simulink model "CurrentSystem2019a"  (R2019a)
settings: Solver=ode23tb  StartTime=0  StopTime=24*365*60*60  RelTol=0.1  EnableMultiTasking=on
PreLoadFcn:
  | power_13NodeTestFeeder_init;
undefined symbols (not defined in the file): ABSOLARCap, ABWindCap, BCSOLARCap, BCWindCap, C_601, C_602, C_603, C_604, C_605, C_606, C_607, ft2km, L_601, L_602, L_603, L_604, L_605, L_606, L_607, MBSOLARCap, MBWindCap, NBSOLARCap, NBWindCap, NLSOLARCap, NLWindCap, NSSOLARCap, NSWindCap, NTSOLARCap, NTWindCap, NUSOLARCap, NUWindCap, ONSOLARCap, ONWindCap, PEISOLARCap, PEIWindCap, QCSOLARCap, QCWindCap, R_601, R_602, R_603, R_604, R_605, R_606, R_607, SKSOLARCap, SKWindCap, T_Disconnect, T_Reconnect, Yearsec, YTSOLARCap, YTWindCap
libraries: powerlib_meascontrol x70, powerlib x67, sps_avr x1, spsDieselMotorModel x1
(part 3 of 3)

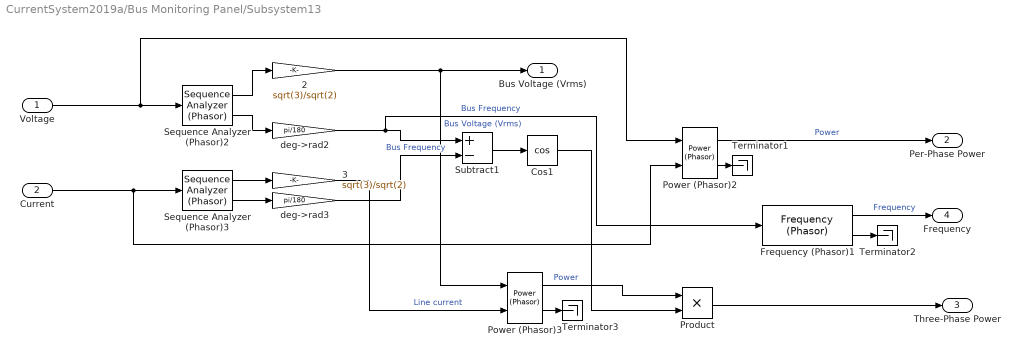
== system CurrentSystem2019a/Bus Monitoring Panel/Subsystem13 ==
  Voltage : Inport
  Current : Inport  Port=2
  " 2" : Gain  Gain=sqrt(3)/sqrt(2)
  " 3" : Gain  Gain=sqrt(3)/sqrt(2)
  Cos1 : Trigonometry  Operator=cos
  Frequency (Phasor)1 : powerlib_meascontrol/Measurements/Frequency (Phasor)  Fn=60  T=0.1
      settings: SourceProductName=Simscape Electrical  SourceProductBaseCode=PS
  Power (Phasor)2 : powerlib_meascontrol/Measurements/Power (Phasor)
      settings: SourceProductName=Simscape Electrical  SourceProductBaseCode=PS
  Power (Phasor)3 : powerlib_meascontrol/Measurements/Power (Phasor)
      settings: SourceProductName=Simscape Electrical  SourceProductBaseCode=PS
  Product : Product
  Sequence Analyzer (Phasor)2 : powerlib_meascontrol/Measurements/Sequence Analyzer (Phasor)  seq=Positive
      settings: SourceProductName=Simscape Electrical  SourceProductBaseCode=PS
  Sequence Analyzer (Phasor)3 : powerlib_meascontrol/Measurements/Sequence Analyzer (Phasor)  seq=Positive
      settings: SourceProductName=Simscape Electrical  SourceProductBaseCode=PS
  Subtract1 : Sum  Inputs=+-
  Terminator1 : Terminator
  Terminator2 : Terminator
  Terminator3 : Terminator
  deg->rad2 : Gain  Gain=pi/180
  deg->rad3 : Gain  Gain=pi/180
  Bus Voltage (Vrms) : Outport  VectorParamsAs1DForOutWhenUnconnected=on
  Per-Phase Power : Outport  Port=2  VectorParamsAs1DForOutWhenUnconnected=on
  Three-Phase Power : Outport  Port=3  VectorParamsAs1DForOutWhenUnconnected=on
  Frequency : Outport  Port=4  VectorParamsAs1DForOutWhenUnconnected=on
  wires:
  Sequence Analyzer (Phasor)2/1 -> " 2"/1
  Sequence Analyzer (Phasor)2/2 -> deg->rad2/1
  Voltage/1 -> Power (Phasor)2/1, Sequence Analyzer (Phasor)2/1
  " 2"/1 -> Power (Phasor)3/1, Bus Voltage (Vrms)/1  "Bus Voltage (Vrms)"
  Sequence Analyzer (Phasor)3/1 -> " 3"/1
  Sequence Analyzer (Phasor)3/2 -> deg->rad3/1
  Current/1 -> Power (Phasor)2/2, Sequence Analyzer (Phasor)3/1
  Subtract1/1 -> Cos1/1
  deg->rad2/1 -> Frequency (Phasor)1/1, Subtract1/1  "Bus Frequency"
  deg->rad3/1 -> Subtract1/2  "Bus Frequency"
  Power (Phasor)2/1 -> Per-Phase Power/1  "Power"
  Power (Phasor)2/2 -> Terminator1/1
  Frequency (Phasor)1/2 -> Terminator2/1
  Frequency (Phasor)1/1 -> Frequency/1  "Frequency"
  " 3"/1 -> Power (Phasor)3/2  "Line current"
  Power (Phasor)3/1 -> Product/1  "Power"
  Cos1/1 -> Product/2
  Power (Phasor)3/2 -> Terminator3/1
  Product/1 -> Three-Phase Power/1

== system CurrentSystem2019a/Bus Monitoring Panel/Subsystem14 ==
  Voltage : Inport
  Current : Inport  Port=2
  Constant : Constant  Value=sqrt(3)
  Cos1 : Trigonometry  Operator=cos
  Product : Product  Inputs=3
  Product2 : Product
  Sequence Analyzer (Phasor)2 : powerlib_meascontrol/Measurements/Sequence Analyzer (Phasor)  seq=Positive
      settings: SourceProductName=Simscape Electrical  SourceProductBaseCode=PS
  Sequence Analyzer (Phasor)3 : powerlib_meascontrol/Measurements/Sequence Analyzer (Phasor)  seq=Positive
      settings: SourceProductName=Simscape Electrical  SourceProductBaseCode=PS
  Subtract1 : Sum  Inputs=+-
  deg->rad2 : Gain  Gain=pi/180
  deg->rad3 : Gain  Gain=pi/180
  Three-Phase Power : Outport  VectorParamsAs1DForOutWhenUnconnected=on
  wires:
  Sequence Analyzer (Phasor)2/1 -> Product2/1
  Product2/1 -> Product/1  "Power"
  Constant/1 -> Product/3
  Current/1 -> Sequence Analyzer (Phasor)3/1
  Sequence Analyzer (Phasor)3/1 -> Product2/2
  Sequence Analyzer (Phasor)3/2 -> deg->rad3/1
  deg->rad2/1 -> Subtract1/1  "Bus Frequency"
  Sequence Analyzer (Phasor)2/2 -> deg->rad2/1
  Subtract1/1 -> Cos1/1
  deg->rad3/1 -> Subtract1/2  "Bus Frequency"
  Voltage/1 -> Sequence Analyzer (Phasor)2/1
  Cos1/1 -> Product/2
  Product/1 -> Three-Phase Power/1

== system CurrentSystem2019a/Bus Monitoring Panel/Subsystem15 ==
  Voltage : Inport
  Current : Inport  Port=2
  Constant : Constant  Value=sqrt(3)
  Cos1 : Trigonometry  Operator=cos
  Product : Product  Inputs=3
  Product2 : Product
  Sequence Analyzer (Phasor)2 : powerlib_meascontrol/Measurements/Sequence Analyzer (Phasor)  seq=Positive
      settings: SourceProductName=Simscape Electrical  SourceProductBaseCode=PS
  Sequence Analyzer (Phasor)3 : powerlib_meascontrol/Measurements/Sequence Analyzer (Phasor)  seq=Positive
      settings: SourceProductName=Simscape Electrical  SourceProductBaseCode=PS
  Subtract1 : Sum  Inputs=+-
  deg->rad2 : Gain  Gain=pi/180
  deg->rad3 : Gain  Gain=pi/180
  Three-Phase Power : Outport  VectorParamsAs1DForOutWhenUnconnected=on
  wires:
  Sequence Analyzer (Phasor)2/1 -> Product2/1
  Product2/1 -> Product/1  "Power"
  Constant/1 -> Product/3
  Current/1 -> Sequence Analyzer (Phasor)3/1
  Sequence Analyzer (Phasor)3/1 -> Product2/2
  Sequence Analyzer (Phasor)3/2 -> deg->rad3/1
  deg->rad2/1 -> Subtract1/1  "Bus Frequency"
  Sequence Analyzer (Phasor)2/2 -> deg->rad2/1
  Subtract1/1 -> Cos1/1
  deg->rad3/1 -> Subtract1/2  "Bus Frequency"
  Voltage/1 -> Sequence Analyzer (Phasor)2/1
  Cos1/1 -> Product/2
  Product/1 -> Three-Phase Power/1

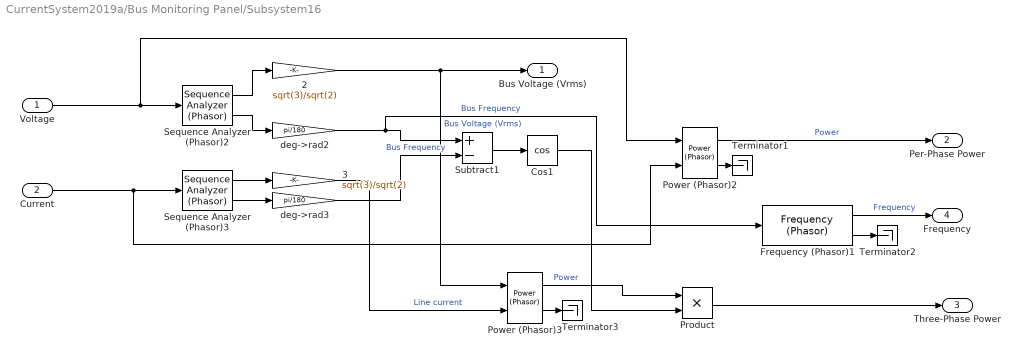
== system CurrentSystem2019a/Bus Monitoring Panel/Subsystem16 ==
  Voltage : Inport
  Current : Inport  Port=2
  " 2" : Gain  Gain=sqrt(3)/sqrt(2)
  " 3" : Gain  Gain=sqrt(3)/sqrt(2)
  Cos1 : Trigonometry  Operator=cos
  Frequency (Phasor)1 : powerlib_meascontrol/Measurements/Frequency (Phasor)  Fn=60  T=0.1
      settings: SourceProductName=Simscape Electrical  SourceProductBaseCode=PS
  Power (Phasor)2 : powerlib_meascontrol/Measurements/Power (Phasor)
      settings: SourceProductName=Simscape Electrical  SourceProductBaseCode=PS
  Power (Phasor)3 : powerlib_meascontrol/Measurements/Power (Phasor)
      settings: SourceProductName=Simscape Electrical  SourceProductBaseCode=PS
  Product : Product
  Sequence Analyzer (Phasor)2 : powerlib_meascontrol/Measurements/Sequence Analyzer (Phasor)  seq=Positive
      settings: SourceProductName=Simscape Electrical  SourceProductBaseCode=PS
  Sequence Analyzer (Phasor)3 : powerlib_meascontrol/Measurements/Sequence Analyzer (Phasor)  seq=Positive
      settings: SourceProductName=Simscape Electrical  SourceProductBaseCode=PS
  Subtract1 : Sum  Inputs=+-
  Terminator1 : Terminator
  Terminator2 : Terminator
  Terminator3 : Terminator
  deg->rad2 : Gain  Gain=pi/180
  deg->rad3 : Gain  Gain=pi/180
  Bus Voltage (Vrms) : Outport  VectorParamsAs1DForOutWhenUnconnected=on
  Per-Phase Power : Outport  Port=2  VectorParamsAs1DForOutWhenUnconnected=on
  Three-Phase Power : Outport  Port=3  VectorParamsAs1DForOutWhenUnconnected=on
  Frequency : Outport  Port=4  VectorParamsAs1DForOutWhenUnconnected=on
  wires:
  Sequence Analyzer (Phasor)2/1 -> " 2"/1
  Sequence Analyzer (Phasor)2/2 -> deg->rad2/1
  Voltage/1 -> Power (Phasor)2/1, Sequence Analyzer (Phasor)2/1
  " 2"/1 -> Power (Phasor)3/1, Bus Voltage (Vrms)/1  "Bus Voltage (Vrms)"
  Sequence Analyzer (Phasor)3/1 -> " 3"/1
  Sequence Analyzer (Phasor)3/2 -> deg->rad3/1
  Current/1 -> Power (Phasor)2/2, Sequence Analyzer (Phasor)3/1
  Subtract1/1 -> Cos1/1
  deg->rad2/1 -> Frequency (Phasor)1/1, Subtract1/1  "Bus Frequency"
  deg->rad3/1 -> Subtract1/2  "Bus Frequency"
  Power (Phasor)2/1 -> Per-Phase Power/1  "Power"
  Power (Phasor)2/2 -> Terminator1/1
  Frequency (Phasor)1/2 -> Terminator2/1
  Frequency (Phasor)1/1 -> Frequency/1  "Frequency"
  " 3"/1 -> Power (Phasor)3/2  "Line current"
  Power (Phasor)3/1 -> Product/1  "Power"
  Cos1/1 -> Product/2
  Power (Phasor)3/2 -> Terminator3/1
  Product/1 -> Three-Phase Power/1

== system CurrentSystem2019a/Bus Monitoring Panel/Subsystem17 ==
  Voltage : Inport
  Current : Inport  Port=2
  Constant : Constant  Value=sqrt(3)
  Cos1 : Trigonometry  Operator=cos
  Product : Product  Inputs=3
  Product2 : Product
  Sequence Analyzer (Phasor)2 : powerlib_meascontrol/Measurements/Sequence Analyzer (Phasor)  seq=Positive
      settings: SourceProductName=Simscape Electrical  SourceProductBaseCode=PS
  Sequence Analyzer (Phasor)3 : powerlib_meascontrol/Measurements/Sequence Analyzer (Phasor)  seq=Positive
      settings: SourceProductName=Simscape Electrical  SourceProductBaseCode=PS
  Subtract1 : Sum  Inputs=+-
  deg->rad2 : Gain  Gain=pi/180
  deg->rad3 : Gain  Gain=pi/180
  Three-Phase Power : Outport  VectorParamsAs1DForOutWhenUnconnected=on
  wires:
  Product/1 -> Three-Phase Power/1
  Product2/1 -> Product/1  "Power"
  Voltage/1 -> Sequence Analyzer (Phasor)2/1
  Sequence Analyzer (Phasor)2/2 -> deg->rad2/1
  Constant/1 -> Product/3
  Cos1/1 -> Product/2
  deg->rad2/1 -> Subtract1/1  "Bus Frequency"
  Subtract1/1 -> Cos1/1
  Current/1 -> Sequence Analyzer (Phasor)3/1
  deg->rad3/1 -> Subtract1/2  "Bus Frequency"
  Sequence Analyzer (Phasor)3/1 -> Product2/2
  Sequence Analyzer (Phasor)2/1 -> Product2/1
  Sequence Analyzer (Phasor)3/2 -> deg->rad3/1

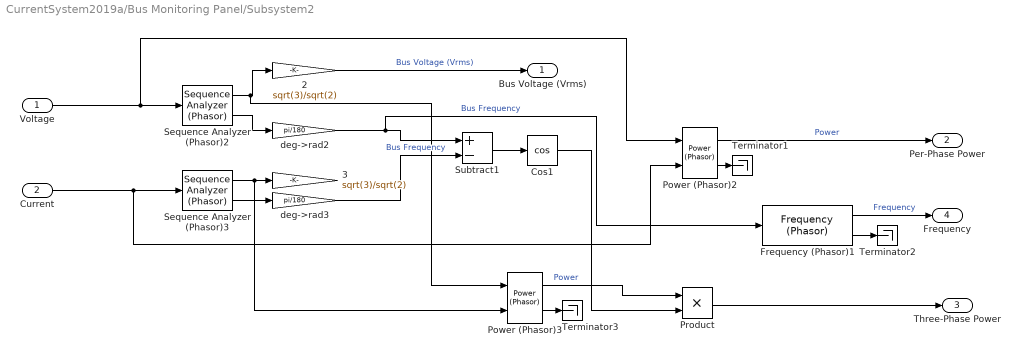
== system CurrentSystem2019a/Bus Monitoring Panel/Subsystem2 ==
  Voltage : Inport
  Current : Inport  Port=2
  " 2" : Gain  Gain=sqrt(3)/sqrt(2)
  " 3" : Gain  Gain=sqrt(3)/sqrt(2)
  Cos1 : Trigonometry  Operator=cos
  Frequency (Phasor)1 : powerlib_meascontrol/Measurements/Frequency (Phasor)  Fn=60  T=0.1
      settings: SourceProductName=Simscape Electrical  SourceProductBaseCode=PS
  Power (Phasor)2 : powerlib_meascontrol/Measurements/Power (Phasor)
      settings: SourceProductName=Simscape Electrical  SourceProductBaseCode=PS
  Power (Phasor)3 : powerlib_meascontrol/Measurements/Power (Phasor)
      settings: SourceProductName=Simscape Electrical  SourceProductBaseCode=PS
  Product : Product
  Sequence Analyzer (Phasor)2 : powerlib_meascontrol/Measurements/Sequence Analyzer (Phasor)  seq=Positive
      settings: SourceProductName=Simscape Electrical  SourceProductBaseCode=PS
  Sequence Analyzer (Phasor)3 : powerlib_meascontrol/Measurements/Sequence Analyzer (Phasor)  seq=Positive
      settings: SourceProductName=Simscape Electrical  SourceProductBaseCode=PS
  Subtract1 : Sum  Inputs=+-
  Terminator1 : Terminator
  Terminator2 : Terminator
  Terminator3 : Terminator
  deg->rad2 : Gain  Gain=pi/180
  deg->rad3 : Gain  Gain=pi/180
  Bus Voltage (Vrms) : Outport  VectorParamsAs1DForOutWhenUnconnected=on
  Per-Phase Power : Outport  Port=2  VectorParamsAs1DForOutWhenUnconnected=on
  Three-Phase Power : Outport  Port=3  VectorParamsAs1DForOutWhenUnconnected=on
  Frequency : Outport  Port=4  VectorParamsAs1DForOutWhenUnconnected=on
  wires:
  Sequence Analyzer (Phasor)2/1 -> Power (Phasor)3/1, " 2"/1
  Sequence Analyzer (Phasor)2/2 -> deg->rad2/1
  Voltage/1 -> Power (Phasor)2/1, Sequence Analyzer (Phasor)2/1
  " 2"/1 -> Bus Voltage (Vrms)/1  "Bus Voltage (Vrms)"
  Sequence Analyzer (Phasor)3/1 -> Power (Phasor)3/2, " 3"/1
  Sequence Analyzer (Phasor)3/2 -> deg->rad3/1
  Current/1 -> Power (Phasor)2/2, Sequence Analyzer (Phasor)3/1
  Subtract1/1 -> Cos1/1
  deg->rad2/1 -> Frequency (Phasor)1/1, Subtract1/1  "Bus Frequency"
  deg->rad3/1 -> Subtract1/2  "Bus Frequency"
  Power (Phasor)2/1 -> Per-Phase Power/1  "Power"
  Power (Phasor)2/2 -> Terminator1/1
  Frequency (Phasor)1/2 -> Terminator2/1
  Frequency (Phasor)1/1 -> Frequency/1  "Frequency"
  Power (Phasor)3/1 -> Product/1  "Power"
  Cos1/1 -> Product/2
  Power (Phasor)3/2 -> Terminator3/1
  Product/1 -> Three-Phase Power/1

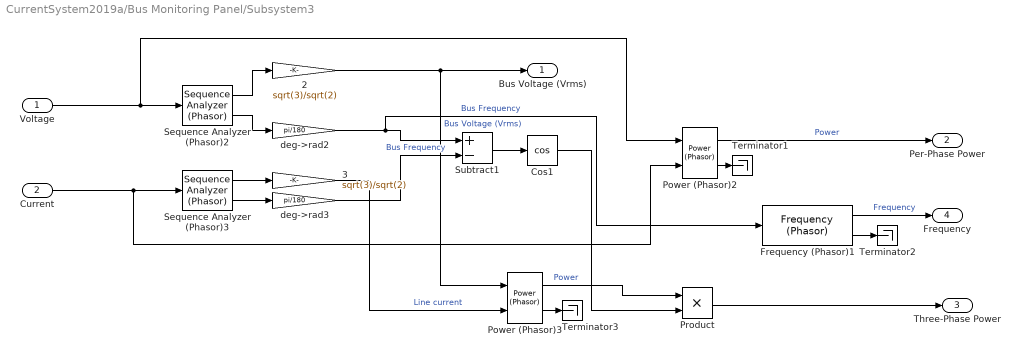
== system CurrentSystem2019a/Bus Monitoring Panel/Subsystem3 ==
  Voltage : Inport
  Current : Inport  Port=2
  " 2" : Gain  Gain=sqrt(3)/sqrt(2)
  " 3" : Gain  Gain=sqrt(3)/sqrt(2)
  Cos1 : Trigonometry  Operator=cos
  Frequency (Phasor)1 : powerlib_meascontrol/Measurements/Frequency (Phasor)  Fn=60  T=0.1
      settings: SourceProductName=Simscape Electrical  SourceProductBaseCode=PS
  Power (Phasor)2 : powerlib_meascontrol/Measurements/Power (Phasor)
      settings: SourceProductName=Simscape Electrical  SourceProductBaseCode=PS
  Power (Phasor)3 : powerlib_meascontrol/Measurements/Power (Phasor)
      settings: SourceProductName=Simscape Electrical  SourceProductBaseCode=PS
  Product : Product
  Sequence Analyzer (Phasor)2 : powerlib_meascontrol/Measurements/Sequence Analyzer (Phasor)  seq=Positive
      settings: SourceProductName=Simscape Electrical  SourceProductBaseCode=PS
  Sequence Analyzer (Phasor)3 : powerlib_meascontrol/Measurements/Sequence Analyzer (Phasor)  seq=Positive
      settings: SourceProductName=Simscape Electrical  SourceProductBaseCode=PS
  Subtract1 : Sum  Inputs=+-
  Terminator1 : Terminator
  Terminator2 : Terminator
  Terminator3 : Terminator
  deg->rad2 : Gain  Gain=pi/180
  deg->rad3 : Gain  Gain=pi/180
  Bus Voltage (Vrms) : Outport  VectorParamsAs1DForOutWhenUnconnected=on
  Per-Phase Power : Outport  Port=2  VectorParamsAs1DForOutWhenUnconnected=on
  Three-Phase Power : Outport  Port=3  VectorParamsAs1DForOutWhenUnconnected=on
  Frequency : Outport  Port=4  VectorParamsAs1DForOutWhenUnconnected=on
  wires:
  Sequence Analyzer (Phasor)2/1 -> " 2"/1
  Sequence Analyzer (Phasor)2/2 -> deg->rad2/1
  Voltage/1 -> Power (Phasor)2/1, Sequence Analyzer (Phasor)2/1
  " 2"/1 -> Power (Phasor)3/1, Bus Voltage (Vrms)/1  "Bus Voltage (Vrms)"
  Sequence Analyzer (Phasor)3/1 -> " 3"/1
  Sequence Analyzer (Phasor)3/2 -> deg->rad3/1
  Current/1 -> Power (Phasor)2/2, Sequence Analyzer (Phasor)3/1
  Subtract1/1 -> Cos1/1
  deg->rad2/1 -> Frequency (Phasor)1/1, Subtract1/1  "Bus Frequency"
  deg->rad3/1 -> Subtract1/2  "Bus Frequency"
  Power (Phasor)2/1 -> Per-Phase Power/1  "Power"
  Power (Phasor)2/2 -> Terminator1/1
  Frequency (Phasor)1/2 -> Terminator2/1
  Frequency (Phasor)1/1 -> Frequency/1  "Frequency"
  " 3"/1 -> Power (Phasor)3/2  "Line current"
  Power (Phasor)3/1 -> Product/1  "Power"
  Cos1/1 -> Product/2
  Power (Phasor)3/2 -> Terminator3/1
  Product/1 -> Three-Phase Power/1

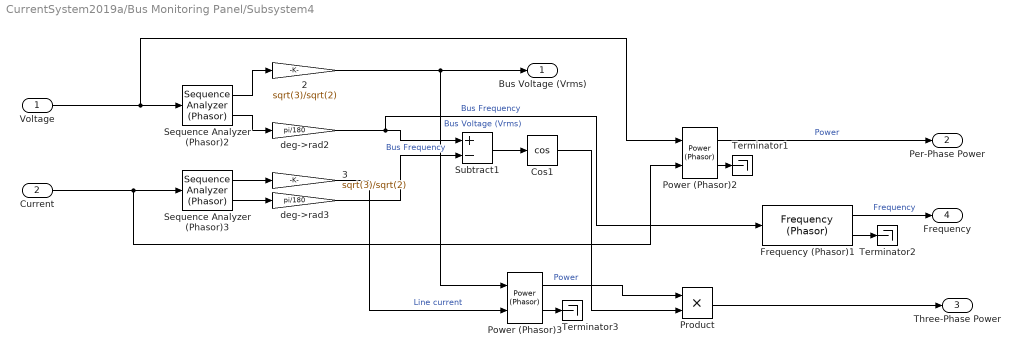
== system CurrentSystem2019a/Bus Monitoring Panel/Subsystem4 ==
  Voltage : Inport
  Current : Inport  Port=2
  " 2" : Gain  Gain=sqrt(3)/sqrt(2)
  " 3" : Gain  Gain=sqrt(3)/sqrt(2)
  Cos1 : Trigonometry  Operator=cos
  Frequency (Phasor)1 : powerlib_meascontrol/Measurements/Frequency (Phasor)  Fn=60  T=0.1
      settings: SourceProductName=Simscape Electrical  SourceProductBaseCode=PS
  Power (Phasor)2 : powerlib_meascontrol/Measurements/Power (Phasor)
      settings: SourceProductName=Simscape Electrical  SourceProductBaseCode=PS
  Power (Phasor)3 : powerlib_meascontrol/Measurements/Power (Phasor)
      settings: SourceProductName=Simscape Electrical  SourceProductBaseCode=PS
  Product : Product
  Sequence Analyzer (Phasor)2 : powerlib_meascontrol/Measurements/Sequence Analyzer (Phasor)  seq=Positive
      settings: SourceProductName=Simscape Electrical  SourceProductBaseCode=PS
  Sequence Analyzer (Phasor)3 : powerlib_meascontrol/Measurements/Sequence Analyzer (Phasor)  seq=Positive
      settings: SourceProductName=Simscape Electrical  SourceProductBaseCode=PS
  Subtract1 : Sum  Inputs=+-
  Terminator1 : Terminator
  Terminator2 : Terminator
  Terminator3 : Terminator
  deg->rad2 : Gain  Gain=pi/180
  deg->rad3 : Gain  Gain=pi/180
  Bus Voltage (Vrms) : Outport  VectorParamsAs1DForOutWhenUnconnected=on
  Per-Phase Power : Outport  Port=2  VectorParamsAs1DForOutWhenUnconnected=on
  Three-Phase Power : Outport  Port=3  VectorParamsAs1DForOutWhenUnconnected=on
  Frequency : Outport  Port=4  VectorParamsAs1DForOutWhenUnconnected=on
  wires:
  Sequence Analyzer (Phasor)2/1 -> " 2"/1
  Sequence Analyzer (Phasor)2/2 -> deg->rad2/1
  Voltage/1 -> Power (Phasor)2/1, Sequence Analyzer (Phasor)2/1
  " 2"/1 -> Power (Phasor)3/1, Bus Voltage (Vrms)/1  "Bus Voltage (Vrms)"
  Sequence Analyzer (Phasor)3/1 -> " 3"/1
  Sequence Analyzer (Phasor)3/2 -> deg->rad3/1
  Current/1 -> Power (Phasor)2/2, Sequence Analyzer (Phasor)3/1
  Subtract1/1 -> Cos1/1
  deg->rad2/1 -> Frequency (Phasor)1/1, Subtract1/1  "Bus Frequency"
  deg->rad3/1 -> Subtract1/2  "Bus Frequency"
  Power (Phasor)2/1 -> Per-Phase Power/1  "Power"
  Power (Phasor)2/2 -> Terminator1/1
  Frequency (Phasor)1/2 -> Terminator2/1
  Frequency (Phasor)1/1 -> Frequency/1  "Frequency"
  " 3"/1 -> Power (Phasor)3/2  "Line current"
  Power (Phasor)3/1 -> Product/1  "Power"
  Cos1/1 -> Product/2
  Power (Phasor)3/2 -> Terminator3/1
  Product/1 -> Three-Phase Power/1

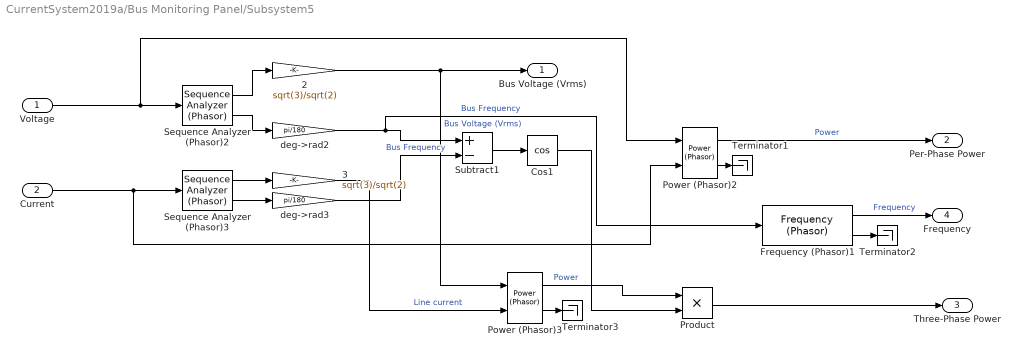
== system CurrentSystem2019a/Bus Monitoring Panel/Subsystem5 ==
  Voltage : Inport
  Current : Inport  Port=2
  " 2" : Gain  Gain=sqrt(3)/sqrt(2)
  " 3" : Gain  Gain=sqrt(3)/sqrt(2)
  Cos1 : Trigonometry  Operator=cos
  Frequency (Phasor)1 : powerlib_meascontrol/Measurements/Frequency (Phasor)  Fn=60  T=0.1
      settings: SourceProductName=Simscape Electrical  SourceProductBaseCode=PS
  Power (Phasor)2 : powerlib_meascontrol/Measurements/Power (Phasor)
      settings: SourceProductName=Simscape Electrical  SourceProductBaseCode=PS
  Power (Phasor)3 : powerlib_meascontrol/Measurements/Power (Phasor)
      settings: SourceProductName=Simscape Electrical  SourceProductBaseCode=PS
  Product : Product
  Sequence Analyzer (Phasor)2 : powerlib_meascontrol/Measurements/Sequence Analyzer (Phasor)  seq=Positive
      settings: SourceProductName=Simscape Electrical  SourceProductBaseCode=PS
  Sequence Analyzer (Phasor)3 : powerlib_meascontrol/Measurements/Sequence Analyzer (Phasor)  seq=Positive
      settings: SourceProductName=Simscape Electrical  SourceProductBaseCode=PS
  Subtract1 : Sum  Inputs=+-
  Terminator1 : Terminator
  Terminator2 : Terminator
  Terminator3 : Terminator
  deg->rad2 : Gain  Gain=pi/180
  deg->rad3 : Gain  Gain=pi/180
  Bus Voltage (Vrms) : Outport  VectorParamsAs1DForOutWhenUnconnected=on
  Per-Phase Power : Outport  Port=2  VectorParamsAs1DForOutWhenUnconnected=on
  Three-Phase Power : Outport  Port=3  VectorParamsAs1DForOutWhenUnconnected=on
  Frequency : Outport  Port=4  VectorParamsAs1DForOutWhenUnconnected=on
  wires:
  Sequence Analyzer (Phasor)2/1 -> " 2"/1
  Sequence Analyzer (Phasor)2/2 -> deg->rad2/1
  Voltage/1 -> Power (Phasor)2/1, Sequence Analyzer (Phasor)2/1
  " 2"/1 -> Power (Phasor)3/1, Bus Voltage (Vrms)/1  "Bus Voltage (Vrms)"
  Sequence Analyzer (Phasor)3/1 -> " 3"/1
  Sequence Analyzer (Phasor)3/2 -> deg->rad3/1
  Current/1 -> Power (Phasor)2/2, Sequence Analyzer (Phasor)3/1
  Subtract1/1 -> Cos1/1
  deg->rad2/1 -> Frequency (Phasor)1/1, Subtract1/1  "Bus Frequency"
  deg->rad3/1 -> Subtract1/2  "Bus Frequency"
  Power (Phasor)2/1 -> Per-Phase Power/1  "Power"
  Power (Phasor)2/2 -> Terminator1/1
  Frequency (Phasor)1/2 -> Terminator2/1
  Frequency (Phasor)1/1 -> Frequency/1  "Frequency"
  " 3"/1 -> Power (Phasor)3/2  "Line current"
  Power (Phasor)3/1 -> Product/1  "Power"
  Cos1/1 -> Product/2
  Power (Phasor)3/2 -> Terminator3/1
  Product/1 -> Three-Phase Power/1

== system CurrentSystem2019a/Bus Monitoring Panel/Subsystem6 ==
  Voltage : Inport
  " 2" : Gain  Gain=sqrt(3)/sqrt(2)
  Frequency (Phasor)1 : powerlib_meascontrol/Measurements/Frequency (Phasor)  Fn=60  T=0.1
      settings: SourceProductName=Simscape Electrical  SourceProductBaseCode=PS
  Sequence Analyzer (Phasor)2 : powerlib_meascontrol/Measurements/Sequence Analyzer (Phasor)  seq=Positive
      settings: SourceProductName=Simscape Electrical  SourceProductBaseCode=PS
  Terminator2 : Terminator
  deg->rad2 : Gain  Gain=pi/180
  Bus Voltage (Vrms) : Outport  VectorParamsAs1DForOutWhenUnconnected=on
  Frequency : Outport  Port=2  VectorParamsAs1DForOutWhenUnconnected=on
  wires:
  Sequence Analyzer (Phasor)2/1 -> " 2"/1
  Sequence Analyzer (Phasor)2/2 -> deg->rad2/1
  Voltage/1 -> Sequence Analyzer (Phasor)2/1
  " 2"/1 -> Bus Voltage (Vrms)/1  "Bus Voltage (Vrms)"
  deg->rad2/1 -> Frequency (Phasor)1/1  "Bus Frequency"
  Frequency (Phasor)1/2 -> Terminator2/1
  Frequency (Phasor)1/1 -> Frequency/1  "Frequency"

== system CurrentSystem2019a/Bus Monitoring Panel/Subsystem7 ==
  Voltage : Inport
  Current : Inport  Port=2
  Constant : Constant  Value=sqrt(3)
  Cos1 : Trigonometry  Operator=cos
  Product : Product  Inputs=3
  Product2 : Product
  Sequence Analyzer (Phasor)2 : powerlib_meascontrol/Measurements/Sequence Analyzer (Phasor)  seq=Positive
      settings: SourceProductName=Simscape Electrical  SourceProductBaseCode=PS
  Sequence Analyzer (Phasor)3 : powerlib_meascontrol/Measurements/Sequence Analyzer (Phasor)  seq=Positive
      settings: SourceProductName=Simscape Electrical  SourceProductBaseCode=PS
  Subtract1 : Sum  Inputs=+-
  deg->rad2 : Gain  Gain=pi/180
  deg->rad3 : Gain  Gain=pi/180
  Three-Phase Power : Outport  VectorParamsAs1DForOutWhenUnconnected=on
  wires:
  Sequence Analyzer (Phasor)2/1 -> Product2/1
  Product2/1 -> Product/1  "Power"
  Constant/1 -> Product/3
  Current/1 -> Sequence Analyzer (Phasor)3/1
  Sequence Analyzer (Phasor)3/1 -> Product2/2
  Sequence Analyzer (Phasor)3/2 -> deg->rad3/1
  deg->rad2/1 -> Subtract1/1  "Bus Frequency"
  Sequence Analyzer (Phasor)2/2 -> deg->rad2/1
  Subtract1/1 -> Cos1/1
  deg->rad3/1 -> Subtract1/2  "Bus Frequency"
  Voltage/1 -> Sequence Analyzer (Phasor)2/1
  Cos1/1 -> Product/2
  Product/1 -> Three-Phase Power/1

== system CurrentSystem2019a/Bus Monitoring Panel/Subsystem8 ==
  Voltage : Inport
  Current : Inport  Port=2
  " 2" : Gain  Gain=sqrt(3)/sqrt(2)
  " 3" : Gain  Gain=sqrt(3)/sqrt(2)
  Cos1 : Trigonometry  Operator=cos
  Frequency (Phasor)1 : powerlib_meascontrol/Measurements/Frequency (Phasor)  Fn=60  T=0.1
      settings: SourceProductName=Simscape Electrical  SourceProductBaseCode=PS
  Power (Phasor)2 : powerlib_meascontrol/Measurements/Power (Phasor)
      settings: SourceProductName=Simscape Electrical  SourceProductBaseCode=PS
  Power (Phasor)3 : powerlib_meascontrol/Measurements/Power (Phasor)
      settings: SourceProductName=Simscape Electrical  SourceProductBaseCode=PS
  Product : Product
  Sequence Analyzer (Phasor)2 : powerlib_meascontrol/Measurements/Sequence Analyzer (Phasor)  seq=Positive
      settings: SourceProductName=Simscape Electrical  SourceProductBaseCode=PS
  Sequence Analyzer (Phasor)3 : powerlib_meascontrol/Measurements/Sequence Analyzer (Phasor)  seq=Positive
      settings: SourceProductName=Simscape Electrical  SourceProductBaseCode=PS
  Subtract1 : Sum  Inputs=+-
  Terminator1 : Terminator
  Terminator2 : Terminator
  Terminator3 : Terminator
  deg->rad2 : Gain  Gain=pi/180
  deg->rad3 : Gain  Gain=pi/180
  Bus Voltage (Vrms) : Outport  VectorParamsAs1DForOutWhenUnconnected=on
  Per-Phase Power : Outport  Port=2  VectorParamsAs1DForOutWhenUnconnected=on
  Three-Phase Power : Outport  Port=3  VectorParamsAs1DForOutWhenUnconnected=on
  Frequency : Outport  Port=4  VectorParamsAs1DForOutWhenUnconnected=on
  wires:
  Sequence Analyzer (Phasor)2/1 -> " 2"/1
  Sequence Analyzer (Phasor)2/2 -> deg->rad2/1
  Voltage/1 -> Power (Phasor)2/1, Sequence Analyzer (Phasor)2/1
  " 2"/1 -> Power (Phasor)3/1, Bus Voltage (Vrms)/1  "Bus Voltage (Vrms)"
  Sequence Analyzer (Phasor)3/1 -> " 3"/1
  Sequence Analyzer (Phasor)3/2 -> deg->rad3/1
  Current/1 -> Power (Phasor)2/2, Sequence Analyzer (Phasor)3/1
  Subtract1/1 -> Cos1/1
  deg->rad2/1 -> Frequency (Phasor)1/1, Subtract1/1  "Bus Frequency"
  deg->rad3/1 -> Subtract1/2  "Bus Frequency"
  Power (Phasor)2/1 -> Per-Phase Power/1  "Power"
  Power (Phasor)2/2 -> Terminator1/1
  Frequency (Phasor)1/2 -> Terminator2/1
  Frequency (Phasor)1/1 -> Frequency/1  "Frequency"
  " 3"/1 -> Power (Phasor)3/2  "Line current"
  Power (Phasor)3/1 -> Product/1  "Power"
  Cos1/1 -> Product/2
  Power (Phasor)3/2 -> Terminator3/1
  Product/1 -> Three-Phase Power/1

== system CurrentSystem2019a/Bus Monitoring Panel/Subsystem9 ==
  Voltage : Inport
  Current : Inport  Port=2
  " 2" : Gain  Gain=sqrt(3)/sqrt(2)
  " 3" : Gain  Gain=sqrt(3)/sqrt(2)
  Cos1 : Trigonometry  Operator=cos
  Frequency (Phasor)1 : powerlib_meascontrol/Measurements/Frequency (Phasor)  Fn=60  T=0.1
      settings: SourceProductName=Simscape Electrical  SourceProductBaseCode=PS
  Power (Phasor)2 : powerlib_meascontrol/Measurements/Power (Phasor)
      settings: SourceProductName=Simscape Electrical  SourceProductBaseCode=PS
  Power (Phasor)3 : powerlib_meascontrol/Measurements/Power (Phasor)
      settings: SourceProductName=Simscape Electrical  SourceProductBaseCode=PS
  Product : Product
  Sequence Analyzer (Phasor)2 : powerlib_meascontrol/Measurements/Sequence Analyzer (Phasor)  seq=Positive
      settings: SourceProductName=Simscape Electrical  SourceProductBaseCode=PS
  Sequence Analyzer (Phasor)3 : powerlib_meascontrol/Measurements/Sequence Analyzer (Phasor)  seq=Positive
      settings: SourceProductName=Simscape Electrical  SourceProductBaseCode=PS
  Subtract1 : Sum  Inputs=+-
  Terminator1 : Terminator
  Terminator2 : Terminator
  Terminator3 : Terminator
  deg->rad2 : Gain  Gain=pi/180
  deg->rad3 : Gain  Gain=pi/180
  Bus Voltage (Vrms) : Outport  VectorParamsAs1DForOutWhenUnconnected=on
  Per-Phase Power : Outport  Port=2  VectorParamsAs1DForOutWhenUnconnected=on
  Three-Phase Power : Outport  Port=3  VectorParamsAs1DForOutWhenUnconnected=on
  Frequency : Outport  Port=4  VectorParamsAs1DForOutWhenUnconnected=on
  wires:
  Sequence Analyzer (Phasor)2/1 -> " 2"/1
  Sequence Analyzer (Phasor)2/2 -> deg->rad2/1
  Voltage/1 -> Power (Phasor)2/1, Sequence Analyzer (Phasor)2/1
  " 2"/1 -> Power (Phasor)3/1, Bus Voltage (Vrms)/1  "Bus Voltage (Vrms)"
  Sequence Analyzer (Phasor)3/1 -> " 3"/1
  Sequence Analyzer (Phasor)3/2 -> deg->rad3/1
  Current/1 -> Power (Phasor)2/2, Sequence Analyzer (Phasor)3/1
  Subtract1/1 -> Cos1/1
  deg->rad2/1 -> Frequency (Phasor)1/1, Subtract1/1  "Bus Frequency"
  deg->rad3/1 -> Subtract1/2  "Bus Frequency"
  Power (Phasor)2/1 -> Per-Phase Power/1  "Power"
  Power (Phasor)2/2 -> Terminator1/1
  Frequency (Phasor)1/2 -> Terminator2/1
  Frequency (Phasor)1/1 -> Frequency/1  "Frequency"
  " 3"/1 -> Power (Phasor)3/2  "Line current"
  Power (Phasor)3/1 -> Product/1  "Power"
  Cos1/1 -> Product/2
  Power (Phasor)3/2 -> Terminator3/1
  Product/1 -> Three-Phase Power/1

== system CurrentSystem2019a/Diesel Generator1/Generator Measures ==
  m : Inport
  Bus Selector : BusSelector  OutputSignals="dq0 components.Stator voltage  vq (pu),dq0 components.Stator voltage  vd (pu)"  OutputAsBus=on
  Bus Selector1 : BusSelector  OutputSignals="Mechanical.Rotor speed  wm  (pu),dq0 components.Field current  ifd (pu)"
  Fcn1 : Fcn  Expr=sqrt(u(1)^2 + u(2)^2)
  Ifd : Outport
  Vt : Outport  Port=2
  wm : Outport  Port=3
  wires:
  Bus Selector1/1 -> wm/1  "<Rotor speed  wm  (pu)>"
  m/1 -> Bus Selector1/1, Bus Selector/1
  Fcn1/1 -> Vt/1
  Bus Selector/1 -> Fcn1/1
  Bus Selector1/2 -> Ifd/1  "<Field current  ifd (pu)>"

== system CurrentSystem2019a/Diesel Generator1/Selected Measurements ==
  m : Inport
  Bus Creator : BusCreator  Inputs=7
  Bus Selector : BusSelector  OutputSignals="Mechanical.Electrical power  Pe (pu),Mechanical.Rotor speed  wm  (pu),Output active power   Peo (pu),Output reactive power  Qeo (pu)"
  to W : Gain  Gain=Pn
  to W1 : Gain  Gain=Pn
  to W2 : Gain  Gain=Pn
  sm : Outport
  wires:
  to W2/1 -> Bus Creator/7  "Reactive Power (W)"
  to W1/1 -> Bus Creator/6  "Active Power (W)"
  Bus Selector/2 -> Bus Creator/3  "<Rotor speed  wm  (pu)>"
  Bus Creator/1 -> sm/1
  to W/1 -> Bus Creator/1  "Electrical Power (W)"
  Bus Selector/3 -> Bus Creator/4, to W1/1  "<Output active power   Peo (pu)>"
  Bus Selector/1 -> to W/1, Bus Creator/2  "<Electrical power  Pe (pu)>"
  Bus Selector/4 -> Bus Creator/5, to W2/1  "<Output reactive power  Qeo (pu)>"
  m/1 -> Bus Selector/1
